simulink model "gm_rx80211a2l_interface"  (R2016a)
settings: Solver=FixedStepDiscrete  SolverMode=SingleTasking  StartTime=0.0  StopTime=46*tpf  RelTol=1e-3
PreLoadFcn:
  | [srx, str, ffv, stx, stb, spi, spl, spq, ntf, cdi, cds] = rx80211a_r0();
InitFcn:
  | if ~exist('srx','var')
  | [srx, str, ffv, stx, stb, spi, spl, spq, ntf, cdi, cds] = rx80211a_r0();
  | end
  | bitrate = 6e6; % 6 Mbits per second
  | crf = 2; % constant redundancy factor (from conv enc)
  | nepsc = 16; % #empty+pilot subcarriers
  | ncps = 16; % #cyclic prefix samples
  | ndbpf = 24; % #data bits per frame
  | ncbpf = ndbpf * crf; % #coded bits per frame
  | nscpf = ncbpf + nepsc; % #subcarriers per frame
  | nspf = nscpf + 16; % #samples per frame
  | tps = 1e-5; %tpf/nspf; % sample time
  | tpf = tps*nspf; %ndbpf/bitrate; % frame time
undefined symbols (not defined in the file): AXI4, cds, Lite, ntf, Radix, srx
libraries: hdlsllib x31, simulink x13, axiinterfacelib x6, commdigbbndpm3 x1, dspxfrm3 x1, commcnvcod2 x1
settings Model: Creator=wchen  LastModifiedBy=bdroz
settings SolverCC: PositivePriorityOrder=on
settings DataIOCC: LimitDataPoints=on  SaveFormat=Array  SaveOutput=off  SignalLogging=off  SaveTime=off
settings OptimizationCC: BlockReduction=off  ConditionallyExecuteInputs=off  ExpressionDepthLimit=2147483647  OptimizeModelRefInitCode=on  LifeSpan=1  MaxStackSize=64
settings DebuggingCC: AlgebraicLoopMsg=error  UnderspecifiedInitializationDetection=Classic  MergeDetectMultiDrivingBlocksExec=none  SolverPrmCheckMsg=warning  SingleTaskRateTransMsg=error  IntegerOverflowMsg=none  ParameterPrecisionLossMsg=none  AllowSymbolicDim=off  StateNameClashWarn=warning
settings HardwareCC: ProdBitPerPointer=32  ProdLargestAtomicInteger=Long  ProdLargestAtomicFloat=Double  ProdWordSize=32  ProdHWDeviceType=ARM Compatible->ARM Cortex  TargetBitPerPointer=64  TargetLongLongMode=on  TargetIntDivRoundTo=Zero  TargetEndianess=LittleEndian  TargetWordSize=64  TargetHWDeviceType=MATLAB Host
settings ModelReferenceCC: PropagateSignalLabelsOutOfModel=off
settings RTWCC: SystemTargetFile=ert.tlc  HardwareBoard=Xilinx Zynq ZC706 evaluation kit  TemplateMakefile=ert_default_tmf  GenerateReport=on  Toolchain=Xilinx Software Development Kit (SDK)  IncludeHyperlinkInReport=on  LaunchReport=on  GenerateTraceInfo=on  GenerateTraceReport=on  GenerateTraceReportSl=on  GenerateTraceReportSf=on  GenerateTraceReportEml=on
settings CodeAppCC: ForceParamTrailComments=on  IgnoreCustomStorageClasses=off  OperatorAnnotations=on  SimulinkDataObjDesc=on  SFDataObjDesc=on  MATLABFcnDesc=on  InsertBlockDesc=on  MATLABSourceComments=on
settings ConfigComp: CovModelRefEnable=Off

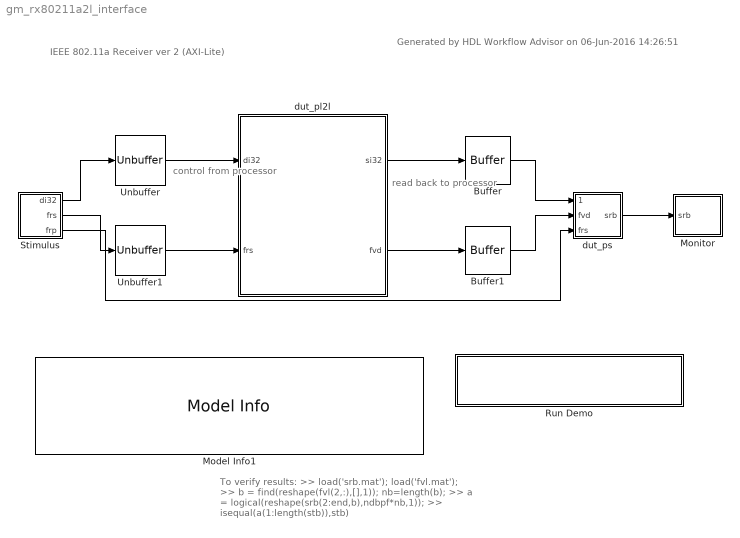
== system gm_rx80211a2l_interface ==
  note: To verify results:
      | >> load('srb.mat'); load('fvl.mat');
      | >> b = find(reshape(fvl(2,:),[],1)); nb=length(b);
      | >> a = logical(reshape(srb(2:end,b),ndbpf*nb,1));
      | >> isequal(a(1:length(stb)),stb)
  note: read back to
      | processor
  note: IEEE 802.11a Receiver ver 2 (AXI-Lite)
  note: control from
      | processor
  note: Generated by HDL Workflow Advisor on 06-Jun-2016 14:26:51
  Buffer : Buffer  N=nspf  TreatMby1Signals=One channel  OutputFrames=off
  Buffer1 : Buffer  N=nspf  TreatMby1Signals=One channel  OutputFrames=off
  Model Info1 : simulink/Model-Wide Utilities/Model Info  Frame=on  DisplayStringWithTags=|  HorizontalTextAlignment=Left  LeftAlignmentValue=0.02  SourceBlockDiagram=gm_rx80211a2l_interface  TagMaxNumber=20
      | This example shows how to use HDL Workflow Advisor to 
      | generate a custom IP core which blink LEDs on FPGA board.
      | 
      | In MATLAB, type the following:
      |   hdladvisor('rx80211a2l/dut_pl2l')
  Monitor : Subsystem  TreatAsAtomicUnit=on
  Run Demo : Subsystem
      settings: OpenFcn=hdladvisor([bdroot, '/dut_pl'])
      mask Display: disp('Launch HDL Workflow Advisor')
  Stimulus : Subsystem
  Unbuffer : Unbuffer  SampleBasedProcessing=Same as frame based
  Unbuffer1 : Unbuffer  SampleBasedProcessing=Same as frame based
  dut_pl2l : Subsystem  TreatAsAtomicUnit=on  mask(AXI4-Lite/AXI4 Interface){}
      mask help:
      | This is an automatically generated subsystem block.
      | This contains the AXI interface blocks that communicate with the dut_pl2l_ip IPCore generated from rx80211a2l/dut_pl2l subsystem.
      mask Display: disp(sprintf('Xilinx Zynq \nAXI Interface'));
  dut_ps : Subsystem
  wires:
  Stimulus/3(frp) -> dut_ps/3(frs)
  Buffer1/1 -> dut_ps/2(fvd)
  dut_pl2l/2(fvd) -> Buffer1/1
  Unbuffer1/1 -> dut_pl2l/2(frs)
  Stimulus/2(frs) -> Unbuffer1/1
  dut_ps/1(srb) -> Monitor/1(srb)
  Buffer/1 -> dut_ps/1(si32)
  Unbuffer/1 -> dut_pl2l/1(di32)
  dut_pl2l/1(si32) -> Buffer/1
  Stimulus/1(di32) -> Unbuffer/1

== system gm_rx80211a2l_interface/Monitor ==
  srb : Inport
  Compare To Constant : simulink/Logic and Bit Operations/Compare To Constant  relop=>  const=uint16(0)  OutDataTypeStr=boolean
  Counter Free-Running : simulink/Sources/Counter Free-Running  NumBits=16  tsamp=tpf
  unpack_int32_into_bool24 : Subsystem
  write_srb_to_file1 : Subsystem
  wires:
  srb/1 -> unpack_int32_into_bool24/1(di32)
  unpack_int32_into_bool24/2(fvd) -> write_srb_to_file1/2(fvl)
  unpack_int32_into_bool24/1(stx) -> write_srb_to_file1/1(srb)
  Compare To Constant/1 -> write_srb_to_file1/Enable
  Counter Free-Running/1 -> Compare To Constant/1

== system gm_rx80211a2l_interface/Run Demo ==

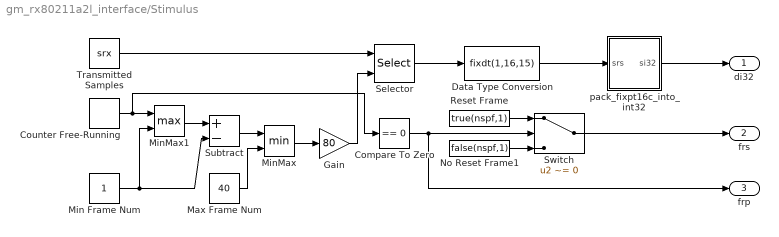
== system gm_rx80211a2l_interface/Stimulus ==
  Compare To Zero : simulink/Logic and Bit Operations/Compare To Zero  relop===  OutDataTypeStr=boolean
  Counter Free-Running : simulink/Sources/Counter Free-Running  NumBits=16  tsamp=tpf
  Data Type Conversion : DataTypeConversion  OutDataTypeStr=fixdt(1,16,15)
  Gain : Gain  Gain=80  OutDataTypeStr=uint16
  Max Frame Num : Constant  Value=40  OutDataTypeStr=uint16  SampleTime=tpf
  Min Frame Num : Constant  OutDataTypeStr=uint16  SampleTime=tpf
  MinMax : MinMax  Inputs=2
  MinMax1 : MinMax  Function=max  Inputs=2
  No Reset Frame1 : Constant  Value=false(nspf,1)  OutDataTypeStr=boolean  SampleTime=tpf
  Reset Frame : Constant  Value=true(nspf,1)  OutDataTypeStr=boolean  SampleTime=tpf
  Selector : Selector  IndexMode=Zero-based  InputPortWidth=3280  IndexOptions=Starting index (port)  Indices=[1 3]  OutputSizes=80
  Subtract : Sum  Inputs=+-
  Switch : Switch  Criteria=u2 ~= 0
  Transmitted Samples : Constant  Value=srx  SampleTime=tpf
  pack_fixpt16c_into_int32 : Subsystem
  di32 : Outport
  frs : Outport  Port=2
  frp : Outport  Port=3
  wires:
  No Reset Frame1/1 -> Switch/3
  Reset Frame/1 -> Switch/1
  Switch/1 -> frs/1
  Compare To Zero/1 -> Switch/2, frp/1
  MinMax1/1 -> Subtract/1
  Subtract/1 -> MinMax/1
  Min Frame Num/1 -> Subtract/2, MinMax1/2
  pack_fixpt16c_into_int32/1(si32) -> di32/1
  Data Type Conversion/1 -> pack_fixpt16c_into_int32/1(srs)
  Selector/1 -> Data Type Conversion/1
  Gain/1 -> Selector/2
  Transmitted Samples/1 -> Selector/1
  MinMax/1 -> Gain/1
  Max Frame Num/1 -> MinMax/2
  Counter Free-Running/1 -> MinMax1/1, Compare To Zero/1

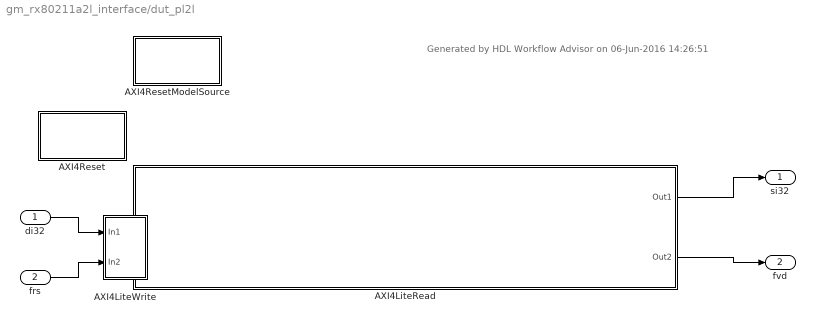
== system gm_rx80211a2l_interface/dut_pl2l ==
  note: Generated by HDL Workflow Advisor on 06-Jun-2016 14:26:51
  di32 : Inport  OutDataTypeStr=uint32
  frs : Inport  Port=2  OutDataTypeStr=boolean
  AXI4LiteRead : Subsystem  Priority=10
  AXI4LiteWrite : Subsystem  Priority=1
  AXI4Reset : Subsystem  mask(System Initialize){ShowInLibBrowser=0}
      mask prompts: ShowInLibBrowser "Simulink:masks:CustCodeMaskParam1_MP"
      settings: CopyFcn=cccopyfcn(gcb)  OpenFcn=ccopenfcn('System Initialize Function')
      mask Help: eval('feval(''rtwprivate'',''rtwhelpview'',''rtw_sys_initialize_block'')');
      mask Display: disp('System\nInitialize');
  AXI4ResetModelSource : Subsystem  mask(Model Source){ShowInLibBrowser=0}
      mask prompts: ShowInLibBrowser "Simulink:masks:CustCodeMaskParam1_MP"
      settings: CopyFcn=cccopyfcn(gcb)  OpenFcn=ccopenfcn('Model Source')
      mask Help: eval('feval(''rtwprivate'',''rtwhelpview'',''rtw_model_source_block'')');
      mask Display: disp('Model\nSource');
  si32 : Outport
  fvd : Outport  Port=2
  wires:
  di32/1 -> AXI4LiteWrite/1(In1)
  frs/1 -> AXI4LiteWrite/2(In2)
  AXI4LiteRead/1(Out1) -> si32/1
  AXI4LiteRead/2(Out2) -> fvd/1

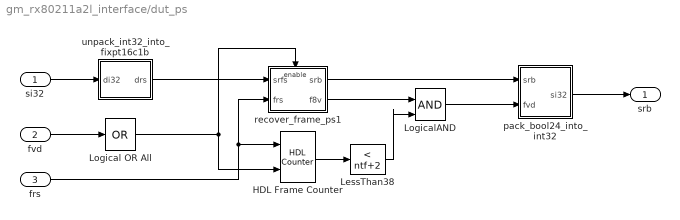
== system gm_rx80211a2l_interface/dut_ps ==
  si32 : Inport
  fvd : Inport  Port=2
  frs : Inport  Port=3
  HDL Frame Counter : hdlsllib/HDL Operations/HDL Counter  CountType=Free running  CountInit=0  CountStep=1  CountMax=25  CountFromType=Initial value  CountFrom=0  CountResetPort=on  CountLoadPort=off  CountEnbPort=on  CountDirPort=off  CountDataType=Unsigned  CountWordLen=8  CountFracLen=0  CountSampTime=1
  LessThan38 : simulink/Logic and Bit Operations/Compare To Constant  relop=<  const=ntf+2  OutDataTypeStr=boolean
  Logical OR All : Logic  Operator=OR  Inputs=1  IconShape=distinctive  AllPortsSameDT=off  OutDataTypeStr=boolean
  LogicalAND : Logic  IconShape=distinctive  AllPortsSameDT=off  OutDataTypeStr=boolean
  pack_bool24_into_int32 : Subsystem
  recover_frame_ps1 : Subsystem  TreatAsAtomicUnit=on
  unpack_int32_into_fixpt16c1b : Subsystem
  srb : Outport
  wires:
  unpack_int32_into_fixpt16c1b/1(drs) -> recover_frame_ps1/1(srfs)
  si32/1 -> unpack_int32_into_fixpt16c1b/1(di32)
  recover_frame_ps1/2(f8v) -> LogicalAND/1
  LogicalAND/1 -> pack_bool24_into_int32/2(fvd)
  LessThan38/1 -> LogicalAND/2
  HDL Frame Counter/1 -> LessThan38/1
  frs/1 -> HDL Frame Counter/1, recover_frame_ps1/2(frs)
  Logical OR All/1 -> HDL Frame Counter/2, recover_frame_ps1/Enable
  pack_bool24_into_int32/1(si32) -> srb/1
  recover_frame_ps1/1(srb) -> pack_bool24_into_int32/1(srb)
  fvd/1 -> Logical OR All/1

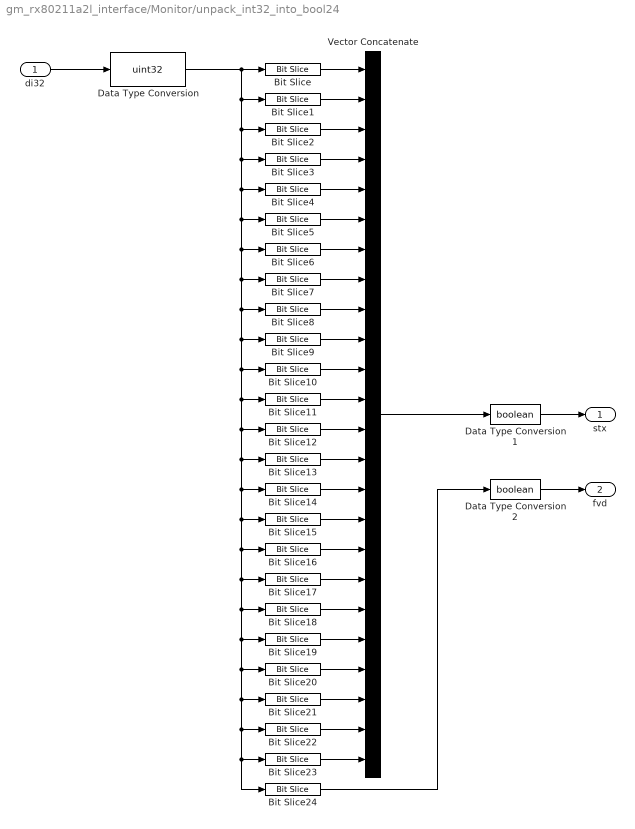
== system gm_rx80211a2l_interface/Monitor/unpack_int32_into_bool24 ==
  di32 : Inport
  Bit Slice : hdlsllib/HDL Operations/Bit Slice  lidx=31  ridx=31
      settings: AttributesFormatString=%<lidx>
  Bit Slice1 : hdlsllib/HDL Operations/Bit Slice  lidx=30  ridx=30
      settings: AttributesFormatString=%<lidx>
  Bit Slice10 : hdlsllib/HDL Operations/Bit Slice  lidx=21  ridx=21
      settings: AttributesFormatString=%<lidx>
  Bit Slice11 : hdlsllib/HDL Operations/Bit Slice  lidx=20  ridx=20
      settings: AttributesFormatString=%<lidx>
  Bit Slice12 : hdlsllib/HDL Operations/Bit Slice  lidx=19  ridx=19
      settings: AttributesFormatString=%<lidx>
  Bit Slice13 : hdlsllib/HDL Operations/Bit Slice  lidx=18  ridx=18
      settings: AttributesFormatString=%<lidx>
  Bit Slice14 : hdlsllib/HDL Operations/Bit Slice  lidx=17  ridx=17
      settings: AttributesFormatString=%<lidx>
  Bit Slice15 : hdlsllib/HDL Operations/Bit Slice  lidx=16  ridx=16
      settings: AttributesFormatString=%<lidx>
  Bit Slice16 : hdlsllib/HDL Operations/Bit Slice  lidx=15  ridx=15
      settings: AttributesFormatString=%<lidx>
  Bit Slice17 : hdlsllib/HDL Operations/Bit Slice  lidx=14  ridx=14
      settings: AttributesFormatString=%<lidx>
  Bit Slice18 : hdlsllib/HDL Operations/Bit Slice  lidx=13  ridx=13
      settings: AttributesFormatString=%<lidx>
  Bit Slice19 : hdlsllib/HDL Operations/Bit Slice  lidx=12  ridx=12
      settings: AttributesFormatString=%<lidx>
  Bit Slice2 : hdlsllib/HDL Operations/Bit Slice  lidx=29  ridx=29
      settings: AttributesFormatString=%<lidx>
  Bit Slice20 : hdlsllib/HDL Operations/Bit Slice  lidx=11  ridx=11
      settings: AttributesFormatString=%<lidx>
  Bit Slice21 : hdlsllib/HDL Operations/Bit Slice  lidx=10  ridx=10
      settings: AttributesFormatString=%<lidx>
  Bit Slice22 : hdlsllib/HDL Operations/Bit Slice  lidx=9  ridx=9
      settings: AttributesFormatString=%<lidx>
  Bit Slice23 : hdlsllib/HDL Operations/Bit Slice  lidx=8  ridx=8
      settings: AttributesFormatString=%<lidx>
  Bit Slice24 : hdlsllib/HDL Operations/Bit Slice  lidx=7  ridx=7
      settings: AttributesFormatString=%<lidx>
  Bit Slice3 : hdlsllib/HDL Operations/Bit Slice  lidx=28  ridx=28
      settings: AttributesFormatString=%<lidx>
  Bit Slice4 : hdlsllib/HDL Operations/Bit Slice  lidx=27  ridx=27
      settings: AttributesFormatString=%<lidx>
  Bit Slice5 : hdlsllib/HDL Operations/Bit Slice  lidx=26  ridx=26
      settings: AttributesFormatString=%<lidx>
  Bit Slice6 : hdlsllib/HDL Operations/Bit Slice  lidx=25  ridx=25
      settings: AttributesFormatString=%<lidx>
  Bit Slice7 : hdlsllib/HDL Operations/Bit Slice  lidx=24  ridx=24
      settings: AttributesFormatString=%<lidx>
  Bit Slice8 : hdlsllib/HDL Operations/Bit Slice  lidx=23  ridx=23
      settings: AttributesFormatString=%<lidx>
  Bit Slice9 : hdlsllib/HDL Operations/Bit Slice  lidx=22  ridx=22
      settings: AttributesFormatString=%<lidx>
  Data Type Conversion : DataTypeConversion  OutDataTypeStr=uint32  ConvertRealWorld=Stored Integer (SI)
  Data Type Conversion1 : DataTypeConversion  OutDataTypeStr=boolean
  Data Type Conversion2 : DataTypeConversion  OutDataTypeStr=boolean
  Vector Concatenate : Concatenate  NumInputs=24
  stx : Outport
  fvd : Outport  Port=2
  wires:
  Data Type Conversion2/1 -> fvd/1
  Data Type Conversion1/1 -> stx/1
  Bit Slice/1 -> Vector Concatenate/1
  Bit Slice1/1 -> Vector Concatenate/2
  Bit Slice2/1 -> Vector Concatenate/3
  Bit Slice3/1 -> Vector Concatenate/4
  Bit Slice4/1 -> Vector Concatenate/5
  Bit Slice5/1 -> Vector Concatenate/6
  Bit Slice6/1 -> Vector Concatenate/7
  Bit Slice7/1 -> Vector Concatenate/8
  Bit Slice8/1 -> Vector Concatenate/9
  Bit Slice9/1 -> Vector Concatenate/10
  Bit Slice10/1 -> Vector Concatenate/11
  Bit Slice11/1 -> Vector Concatenate/12
  Bit Slice12/1 -> Vector Concatenate/13
  Bit Slice13/1 -> Vector Concatenate/14
  Bit Slice14/1 -> Vector Concatenate/15
  Bit Slice15/1 -> Vector Concatenate/16
  Bit Slice16/1 -> Vector Concatenate/17
  Bit Slice17/1 -> Vector Concatenate/18
  Bit Slice18/1 -> Vector Concatenate/19
  Bit Slice19/1 -> Vector Concatenate/20
  Bit Slice20/1 -> Vector Concatenate/21
  Bit Slice21/1 -> Vector Concatenate/22
  Bit Slice22/1 -> Vector Concatenate/23
  Bit Slice23/1 -> Vector Concatenate/24
  Data Type Conversion/1 -> Bit Slice/1, Bit Slice6/1, Bit Slice10/1, Bit Slice14/1, Bit Slice16/1, Bit Slice22/1, Bit Slice23/1, Bit Slice24/1, Bit Slice21/1, Bit Slice20/1, Bit Slice19/1, Bit Slice18/1, Bit Slice17/1, Bit Slice15/1, Bit Slice13/1, Bit Slice12/1, Bit Slice11/1, Bit Slice9/1, Bit Slice8/1, Bit Slice7/1, Bit Slice5/1, Bit Slice4/1, Bit Slice3/1, Bit Slice2/1, Bit Slice1/1
  Bit Slice24/1 -> Data Type Conversion2/1
  Vector Concatenate/1 -> Data Type Conversion1/1
  di32/1 -> Data Type Conversion/1

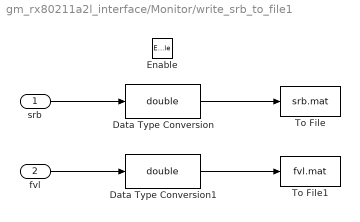
== system gm_rx80211a2l_interface/Monitor/write_srb_to_file1 ==
  srb : Inport
  fvl : Inport  Port=2
  Enable : EnablePort
  Data Type Conversion : DataTypeConversion  OutDataTypeStr=double
  Data Type Conversion1 : DataTypeConversion  OutDataTypeStr=double
  To File : ToFile  Filename=srb.mat  MatrixName=srb  SampleTime=tpf
  To File1 : ToFile  Filename=fvl.mat  MatrixName=fvl  SampleTime=tpf
  wires:
  Data Type Conversion/1 -> To File/1
  srb/1 -> Data Type Conversion/1
  Data Type Conversion1/1 -> To File1/1
  fvl/1 -> Data Type Conversion1/1

== system gm_rx80211a2l_interface/Stimulus/pack_fixpt16c_into_int32 ==
  srs : Inport
  Bit Concat : hdlsllib/HDL Operations/Bit Concat  numInputs=2
  Complex to Real-Imag : ComplexToRealImag
  si32 : Outport
  wires:
  Complex to Real-Imag/2 -> Bit Concat/2
  Bit Concat/1 -> si32/1
  Complex to Real-Imag/1 -> Bit Concat/1
  srs/1 -> Complex to Real-Imag/1

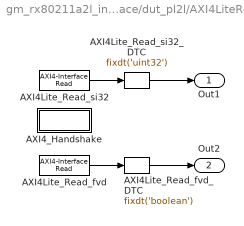
== system gm_rx80211a2l_interface/dut_pl2l/AXI4LiteRead ==
  AXI4Lite_Read_fvd : axiinterfacelib/AXI4-Interface Read  Priority=3  AXIInterfaceType=AXI4-Lite  DeviceName=/dev/mwipcore  RegisterOffset=hex2dec('10C')  DataLength=4096  DataType=uint32  SampleTime=1e-05  blockPlatform=ZYNQ  SimulateUsing=Interpreted Execution
  AXI4Lite_Read_fvd_DTC : DataTypeConversion  OutDataTypeStr=fixdt('boolean')  ConvertRealWorld=Stored Integer (SI)
  AXI4Lite_Read_si32 : axiinterfacelib/AXI4-Interface Read  Priority=2  AXIInterfaceType=AXI4-Lite  DeviceName=/dev/mwipcore  RegisterOffset=hex2dec('108')  DataLength=4096  DataType=uint32  SampleTime=1e-05  blockPlatform=ZYNQ  SimulateUsing=Interpreted Execution
  AXI4Lite_Read_si32_DTC : DataTypeConversion  OutDataTypeStr=fixdt('uint32')  ConvertRealWorld=Stored Integer (SI)
  AXI4_Handshake : Subsystem  Priority=1  mask(AXI4-Lite/AXI4 Handshake){blockPlatform=ZYNQ}
      mask prompts: blockPlatform "Mask Parameter 1:"
      mask help:
      | This is an automatically generated block.
      | It synchronizes the data between ARM and FPGA on AXI4-Lite/AXI4 interface.
      |
      | This block writes the FPGA Strobe signal to indicate that the data from ARM on AXI4-Lite/AXI4 interface is valid.
      |
      | It waits until the FPGA Ready signal is 1 (logic-HIGH), which shows that data from FPGA on AXI4-Lite/AXI4 interface is valid.
      mask Display:
      | color('blue');
      | text(0.67, 0.87, 'ZYNQ', 'horizontalAlignment', 'left');
  Out1 : Outport
  Out2 : Outport  Port=2
  wires:
  AXI4Lite_Read_si32/1 -> AXI4Lite_Read_si32_DTC/1
  AXI4Lite_Read_si32_DTC/1 -> Out1/1
  AXI4Lite_Read_fvd/1 -> AXI4Lite_Read_fvd_DTC/1
  AXI4Lite_Read_fvd_DTC/1 -> Out2/1

== system gm_rx80211a2l_interface/dut_pl2l/AXI4LiteWrite ==
  In1 : Inport
  In2 : Inport  Port=2
  AXI4Lite_Write_di32 : axiinterfacelib/AXI4-Interface Write  Priority=1  AXIInterfaceType=AXI4-Lite  DeviceName=/dev/mwipcore  RegisterOffset=hex2dec('100')  blockPlatform=ZYNQ  SimulateUsing=Interpreted execution
  AXI4Lite_Write_di32_DTC : DataTypeConversion  OutDataTypeStr=uint32  ConvertRealWorld=Stored Integer (SI)
  AXI4Lite_Write_frs : axiinterfacelib/AXI4-Interface Write  Priority=2  AXIInterfaceType=AXI4-Lite  DeviceName=/dev/mwipcore  RegisterOffset=hex2dec('104')  blockPlatform=ZYNQ  SimulateUsing=Interpreted execution
  AXI4Lite_Write_frs_DTC : DataTypeConversion  OutDataTypeStr=uint32  ConvertRealWorld=Stored Integer (SI)
  wires:
  AXI4Lite_Write_di32_DTC/1 -> AXI4Lite_Write_di32/1
  AXI4Lite_Write_frs_DTC/1 -> AXI4Lite_Write_frs/1
  In2/1 -> AXI4Lite_Write_frs_DTC/1
  In1/1 -> AXI4Lite_Write_di32_DTC/1

== system gm_rx80211a2l_interface/dut_pl2l/AXI4Reset ==

== system gm_rx80211a2l_interface/dut_pl2l/AXI4ResetModelSource ==

== system gm_rx80211a2l_interface/dut_ps/pack_bool24_into_int32 ==
  srb : Inport
  fvd : Inport  Port=2
  Bit Concat : hdlsllib/HDL Operations/Bit Concat  numInputs=1
  Constant 7 False Bits : Constant  Value=false(7,1)  OutDataTypeStr=boolean  SampleTime=tpf
  Data Type Conversion : DataTypeConversion  OutDataTypeStr=uint32  ConvertRealWorld=Stored Integer (SI)
  Vector Concatenate : Concatenate  NumInputs=3
  si32 : Outport
  wires:
  Bit Concat/1 -> Data Type Conversion/1
  Data Type Conversion/1 -> si32/1
  Constant 7 False Bits/1 -> Vector Concatenate/3
  fvd/1 -> Vector Concatenate/2
  srb/1 -> Vector Concatenate/1
  Vector Concatenate/1 -> Bit Concat/1

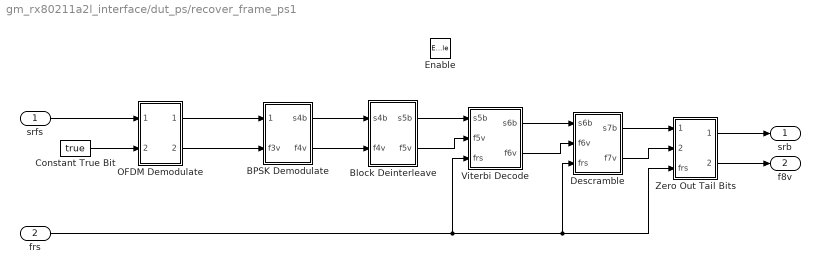
== system gm_rx80211a2l_interface/dut_ps/recover_frame_ps1 ==
  srfs : Inport
  frs : Inport  Port=2
  Enable : EnablePort
  BPSK Demodulate : Subsystem
  Block Deinterleave : Subsystem
  Constant True Bit : Constant  Value=true  OutDataTypeStr=boolean  SampleTime=tpf
  Descramble : Subsystem
  OFDM Demodulate : Subsystem
  Viterbi Decode : Subsystem
  Zero Out Tail Bits : Subsystem
  srb : Outport  InitialOutput=0
  f8v : Outport  Port=2  InitialOutput=0
  wires:
  srfs/1 -> OFDM Demodulate/1(d0s)
  Zero Out Tail Bits/2(f8v) -> f8v/1
  Descramble/2(f7v) -> Zero Out Tail Bits/2(f7v)
  Viterbi Decode/2(f6v) -> Descramble/2(f6v)
  Block Deinterleave/2(f5v) -> Viterbi Decode/2(f5v)
  BPSK Demodulate/2(f4v) -> Block Deinterleave/2(f4v)
  OFDM Demodulate/2(f3v) -> BPSK Demodulate/2(f3v)
  Constant True Bit/1 -> OFDM Demodulate/2(f0v)
  Zero Out Tail Bits/1(s8b) -> srb/1
  Descramble/1(s7b) -> Zero Out Tail Bits/1(s7b)
  Viterbi Decode/1(s6b) -> Descramble/1(s6b)
  Block Deinterleave/1(s5b) -> Viterbi Decode/1(s5b)
  BPSK Demodulate/1(s4b) -> Block Deinterleave/1(s4b)
  OFDM Demodulate/1(d3m) -> BPSK Demodulate/1(d3m)
  frs/1 -> Viterbi Decode/3(frs), Zero Out Tail Bits/3(frs), Descramble/3(frs)

== system gm_rx80211a2l_interface/dut_ps/unpack_int32_into_fixpt16c1b ==
  di32 : Inport
  Data Type Conversion : DataTypeConversion  OutDataTypeStr=fixdt(1,16,15)  ConvertRealWorld=Stored Integer (SI)
      settings: AttributesFormatString=%<OutDataTypeStr>
  Data Type Conversion1 : DataTypeConversion  OutDataTypeStr=fixdt(1,16,15)  ConvertRealWorld=Stored Integer (SI)
      settings: AttributesFormatString=%<OutDataTypeStr>
  Extract Bits : simulink/Logic and Bit Operations/Extract Bits  bitsToExtract=Upper half  numBits=8  bitIdxRange=[0 7]  outScalingMode=Preserve fixed-point scaling
  Extract Bits1 : simulink/Logic and Bit Operations/Extract Bits  bitsToExtract=Lower half  numBits=8  bitIdxRange=[0 7]  outScalingMode=Preserve fixed-point scaling
  Real-Imag to Complex : RealImagToComplex
  drs : Outport
  wires:
  Data Type Conversion1/1 -> Real-Imag to Complex/2
  Data Type Conversion/1 -> Real-Imag to Complex/1
  Extract Bits1/1 -> Data Type Conversion1/1
  Real-Imag to Complex/1 -> drs/1
  Extract Bits/1 -> Data Type Conversion/1
  di32/1 -> Extract Bits/1, Extract Bits1/1

== system gm_rx80211a2l_interface/dut_pl2l/AXI4LiteRead/AXI4_Handshake ==
  AXI4_Write_FPGA_STROBE : axiinterfacelib/AXI4-Interface Write  Priority=1  AXIInterfaceType=AXI4-Lite  DeviceName=/dev/mwipcore  RegisterOffset=hex2dec('8')  blockPlatform=ZYNQ  SimulateUsing=Interpreted execution
  Constant : Constant  OutDataTypeStr=uint32
  WhileIteratorSubsystem : Subsystem  Priority=10  TreatAsAtomicUnit=on
  wires:
  Constant/1 -> AXI4_Write_FPGA_STROBE/1

== system gm_rx80211a2l_interface/dut_ps/recover_frame_ps1/BPSK Demodulate ==
  d3m : Inport
  f3v : Inport  Port=2
  BPSK Demodulator Baseband : commdigbbndpm3/BPSK Demodulator Baseband  DecType=Hard decision  VarSource=Dialog  Variance=1  Ph=0  outDtype=boolean  derotateFactorWordLen=16  derotateFactorDataTypeStr=Inherit: Same word length as input  derotateFactorLastDataTypeStr=Inherit: Same word length as input
  Logical NOT : Logic  Operator=NOT  IconShape=distinctive  AllPortsSameDT=off  OutDataTypeStr=boolean
  s4b : Outport
  f4v : Outport  Port=2
  wires:
  f3v/1 -> f4v/1
  BPSK Demodulator Baseband/1 -> Logical NOT/1
  Logical NOT/1 -> s4b/1
  d3m/1 -> BPSK Demodulator Baseband/1

== system gm_rx80211a2l_interface/dut_ps/recover_frame_ps1/Block Deinterleave ==
  s4b : Inport
  f4v : Inport  Port=2
  block_deinterleave : Selector  IndexMode=Zero-based  InputPortWidth=48  IndexOptions=Index vector (dialog)  Indices=cdi  OutputSizes=1
  s5b : Outport
  f5v : Outport  Port=2
  wires:
  f4v/1 -> f5v/1
  block_deinterleave/1 -> s5b/1
  s4b/1 -> block_deinterleave/1

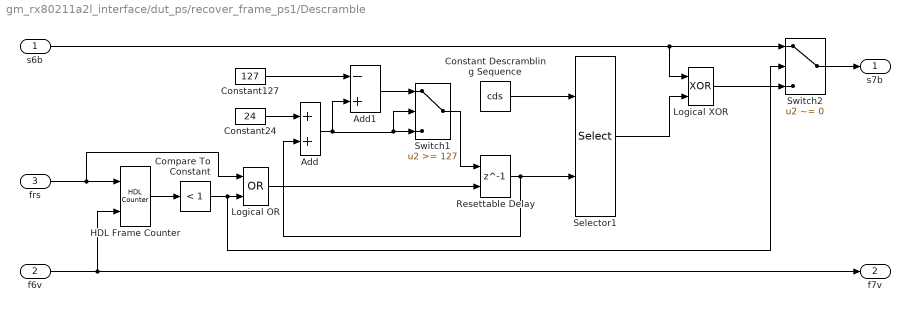
== system gm_rx80211a2l_interface/dut_ps/recover_frame_ps1/Descramble ==
  s6b : Inport
  f6v : Inport  Port=2
  frs : Inport  Port=3
  Add : Sum  OutDataTypeStr=uint8
  Add1 : Sum  Inputs=-+  OutDataTypeStr=uint8
  Compare To Constant : simulink/Logic and Bit Operations/Compare To Constant  relop=<  const=1  OutDataTypeStr=boolean
  Constant Descrambling Sequence : Constant  Value=cds  OutDataTypeStr=boolean  SampleTime=tpf
  Constant127 : Constant  Value=127  OutDataTypeStr=uint8  SampleTime=tpf
  Constant24 : Constant  Value=24  OutDataTypeStr=uint8  SampleTime=tpf
  HDL Frame Counter : hdlsllib/HDL Operations/HDL Counter  CountType=Free running  CountInit=0  CountStep=1  CountMax=23  CountFromType=Initial value  CountFrom=0  CountResetPort=on  CountLoadPort=off  CountEnbPort=on  CountDirPort=off  CountDataType=Unsigned  CountWordLen=16  CountFracLen=0  CountSampTime=tpf
  Logical OR : Logic  Operator=OR  IconShape=distinctive  AllPortsSameDT=off  OutDataTypeStr=boolean
  Logical XOR : Logic  Operator=XOR  IconShape=distinctive  AllPortsSameDT=off  OutDataTypeStr=boolean
  Resettable Delay : Delay  DelayLength=1  InitialCondition=uint8(0)  ExternalReset=Level  SampleTime=tpf
      settings: InputPortMap=u0,r5
  Selector1 : Selector  IndexMode=Zero-based  InputPortWidth=254  IndexOptions=Starting index (port)  Indices=[1 3]  OutputSizes=24
  Switch1 : Switch  Threshold=127
  Switch2 : Switch  Criteria=u2 ~= 0
  s7b : Outport
  f7v : Outport  Port=2
  wires:
  Switch2/1 -> s7b/1
  Logical XOR/1 -> Switch2/3
  Logical OR/1 -> Resettable Delay/2
  Constant127/1 -> Add1/1
  Add1/1 -> Switch1/1
  Add/1 -> Switch1/3, Switch1/2, Add1/2
  Switch1/1 -> Resettable Delay/1
  Constant24/1 -> Add/1
  Selector1/1 -> Logical XOR/2
  Constant Descrambling Sequence/1 -> Selector1/1
  Resettable Delay/1 -> Selector1/2, Add/2
  Compare To Constant/1 -> Logical OR/2, Switch2/2
  frs/1 -> HDL Frame Counter/1, Logical OR/1
  s6b/1 -> Logical XOR/1, Switch2/1
  f6v/1 -> f7v/1, HDL Frame Counter/2
  HDL Frame Counter/1 -> Compare To Constant/1

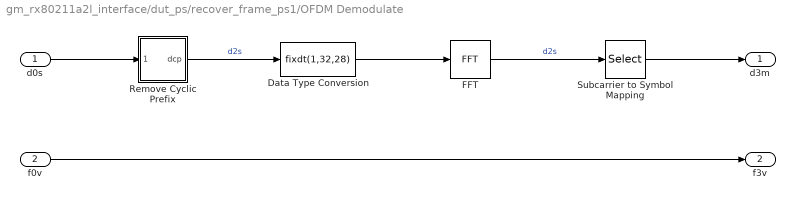
== system gm_rx80211a2l_interface/dut_ps/recover_frame_ps1/OFDM Demodulate ==
  d0s : Inport
  f0v : Inport  Port=2
  Data Type Conversion : DataTypeConversion  OutDataTypeStr=fixdt(1,32,28)
      settings: AttributesFormatString=%<OutDataTypeStr>
  FFT : dspxfrm3/FFT  FFTImplementation=Radix-2  CompMethod=Table lookup  TableOpt=NEW  TableOptActive=Speed  BitRevOrder=off  Normalize=off  InheritFFTLength=off  FFTLength=64  WrapInput=off  roundingMode=Floor  overflowMode=on  firstCoeffMode=Specify word length  firstCoeffWordLength=32  firstCoeffFracLength=15  firstCoeffDataTypeStr=fixdt(1,32)  firstCoeffLastDataTypeStr=fixdt(1,32)  prodOutputMode=Binary point scaling  prodOutputWordLength=32  prodOutputFracLength=28  prodOutputDataTypeStr=fixdt(1,32,28)  prodOutputLastDataTypeStr=fixdt(1,32,28)  accumMode=Binary point scaling  accumWordLength=32  accumFracLength=28  accumDataTypeStr=fixdt(1,32,28)  accumLastDataTypeStr=fixdt(1,32,28)  outputMin=[]  outputMax=[]
  Remove Cyclic Prefix : Subsystem
  Subcarrier to Symbol Mapping : Selector  IndexMode=Zero-based  InputPortWidth=64  IndexOptions=Index vector (dialog)  Indices=[38:42, 44:56, 58:63, 1:6, 8:20, 22:26]  OutputSizes=1
  d3m : Outport
  f3v : Outport  Port=2
  wires:
  Data Type Conversion/1 -> FFT/1
  f0v/1 -> f3v/1
  Remove Cyclic Prefix/1(dcp) -> Data Type Conversion/1  "d2s"
  Subcarrier to Symbol Mapping/1 -> d3m/1
  d0s/1 -> Remove Cyclic Prefix/1(drfs)
  FFT/1 -> Subcarrier to Symbol Mapping/1  "d2s"

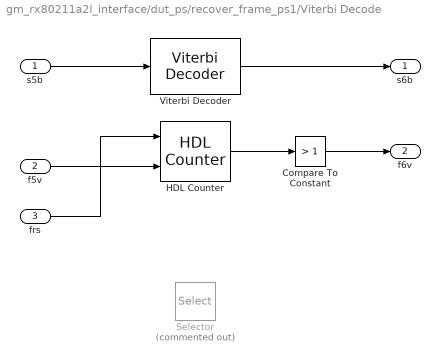
== system gm_rx80211a2l_interface/dut_ps/recover_frame_ps1/Viterbi Decode ==
  s5b : Inport
  f5v : Inport  Port=2
  frs : Inport  Port=3
  Compare To Constant : simulink/Logic and Bit Operations/Compare To Constant  relop=>  const=1  OutDataTypeStr=boolean
  HDL Counter : hdlsllib/HDL Operations/HDL Counter  CountType=Free running  CountInit=0  CountStep=1  CountMax=25  CountFromType=Initial value  CountFrom=0  CountResetPort=on  CountLoadPort=off  CountEnbPort=on  CountDirPort=off  CountDataType=Unsigned  CountWordLen=16  CountFracLen=0  CountSampTime=1
  Selector : Selector  Commented=on  IndexMode=Zero-based  InputPortWidth=48  IndexOptions=Starting index (dialog)  Indices=0  OutputSizes=24
  Viterbi Decoder : commcnvcod2/Viterbi Decoder  trellis=poly2trellis(7, [133,171])  isPunctured=off  punctureVector=[1; 1; 0; 1; 0; 1]  erasures=off  dectype=Hard decision  nsdecb=4  runSigValErrCheck=off  tbdepth=48  opmode=Continuous  reset=off  delayedResetAction=on  smWordLength=16  outDataType=boolean
  s6b : Outport
  f6v : Outport  Port=2
  wires:
  Compare To Constant/1 -> f6v/1
  HDL Counter/1 -> Compare To Constant/1
  f5v/1 -> HDL Counter/2
  frs/1 -> HDL Counter/1
  s5b/1 -> Viterbi Decoder/1
  Viterbi Decoder/1 -> s6b/1

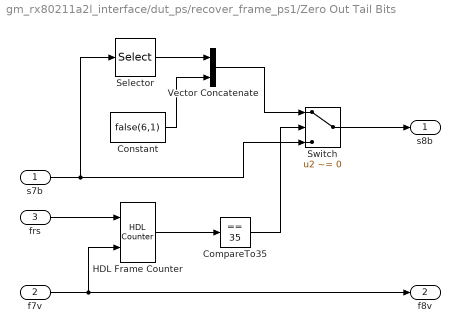
== system gm_rx80211a2l_interface/dut_ps/recover_frame_ps1/Zero Out Tail Bits ==
  s7b : Inport
  f7v : Inport  Port=2
  frs : Inport  Port=3
  CompareTo35 : simulink/Logic and Bit Operations/Compare To Constant  relop===  const=35  OutDataTypeStr=boolean
  Constant : Constant  Value=false(6,1)  OutDataTypeStr=boolean  SampleTime=tpf
  HDL Frame Counter : hdlsllib/HDL Operations/HDL Counter  CountType=Free running  CountInit=0  CountStep=1  CountMax=25  CountFromType=Initial value  CountFrom=0  CountResetPort=on  CountLoadPort=off  CountEnbPort=on  CountDirPort=off  CountDataType=Unsigned  CountWordLen=16  CountFracLen=0  CountSampTime=tpf
  Selector : Selector  IndexMode=Zero-based  InputPortWidth=24  IndexOptions=Index vector (dialog)  Indices=0:17  OutputSizes=1
  Switch : Switch  Criteria=u2 ~= 0  Threshold=36
  Vector Concatenate : Concatenate
  s8b : Outport
  f8v : Outport  Port=2
  wires:
  CompareTo35/1 -> Switch/2
  f7v/1 -> f8v/1, HDL Frame Counter/2
  frs/1 -> HDL Frame Counter/1
  Selector/1 -> Vector Concatenate/1
  Constant/1 -> Vector Concatenate/2
  s7b/1 -> Switch/3, Selector/1
  Switch/1 -> s8b/1
  Vector Concatenate/1 -> Switch/1
  HDL Frame Counter/1 -> CompareTo35/1

== system gm_rx80211a2l_interface/dut_pl2l/AXI4LiteRead/AXI4_Handshake/WhileIteratorSubsystem ==
  AXI4_Read_FPGA_READY : axiinterfacelib/AXI4-Interface Read  Priority=1  AXIInterfaceType=AXI4-Lite  DeviceName=/dev/mwipcore  RegisterOffset=hex2dec('C')  DataLength=4096  DataType=uint32  SampleTime=-1  blockPlatform=ZYNQ  SimulateUsing=Interpreted Execution
  Compare_To_Zero : simulink/Logic and Bit Operations/Compare To Zero  relop===  OutDataTypeStr=boolean
  Constant_SimMode : Constant  OutDataTypeStr=uint32
  EnvController : simulink/Signal Routing/Environment Controller
  While Iterator : WhileIterator  MaxIters=-1  WhileBlockType=do-while  ResetStates=reset
  wires:
  Constant_SimMode/1 -> EnvController/1
  AXI4_Read_FPGA_READY/1 -> EnvController/2
  EnvController/1 -> Compare_To_Zero/1
  Compare_To_Zero/1 -> While Iterator/1

== system gm_rx80211a2l_interface/dut_ps/recover_frame_ps1/OFDM Demodulate/Remove Cyclic Prefix ==
  drfs : Inport
  Selector : Selector  IndexMode=Zero-based  InputPortWidth=80  IndexOptions=Index vector (dialog)  Indices=16:79  OutputSizes=1
  dcp : Outport
  wires:
  drfs/1 -> Selector/1
  Selector/1 -> dcp/1
